simulink model "LQR_Kalman_Hardware"  (R2018b)
settings: Solver=FixedStepAuto  StartTime=0.0  StopTime=inf  FixedStep=0.002  RelTol=1e-3  EnableMultiTasking=on
undefined symbols (not defined in the file): HIL, K_lqr, qc_get_step_size
libraries: quarc_library x3, simulink x1, cstblocks x1
settings Model: SimulationMode=external  ExtModeTrigDuration=10000  Creator=ACSI-MLC  LastModifiedBy=ACSI-MLC
settings SolverCC: PositivePriorityOrder=on
settings RTWCC: SystemTargetFile=quarc_win64.tlc  TemplateMakefile=quarc_default_tmf  Description=QUARC Win64 Target
settings STFCustomTargetCC: TargetPreCompLibLocation=C:\PROGRA~3\QUARC\lib\2018b\win64\release  TargetLangStandard=C99 (ISO)  ConcurrentExecutionCompliant=on  GRTInterface=on  SystemTargetFile=quarc_win64.tlc
settings GRTTargetCC: TargetPreCompLibLocation=C:\PROGRA~3\QUARC\lib\2018b\win64\release  ParMdlRefBuildCompliant=off  CompOptLevelCompliant=off  CombineOutputUpdateFcns=off  MatFileLogging=off  CPPClassGenCompliant=off  GRTInterface=on  UseToolchainInfoCompliant=off  ExtMode=on  ExtModeMexFile=quarc_comm

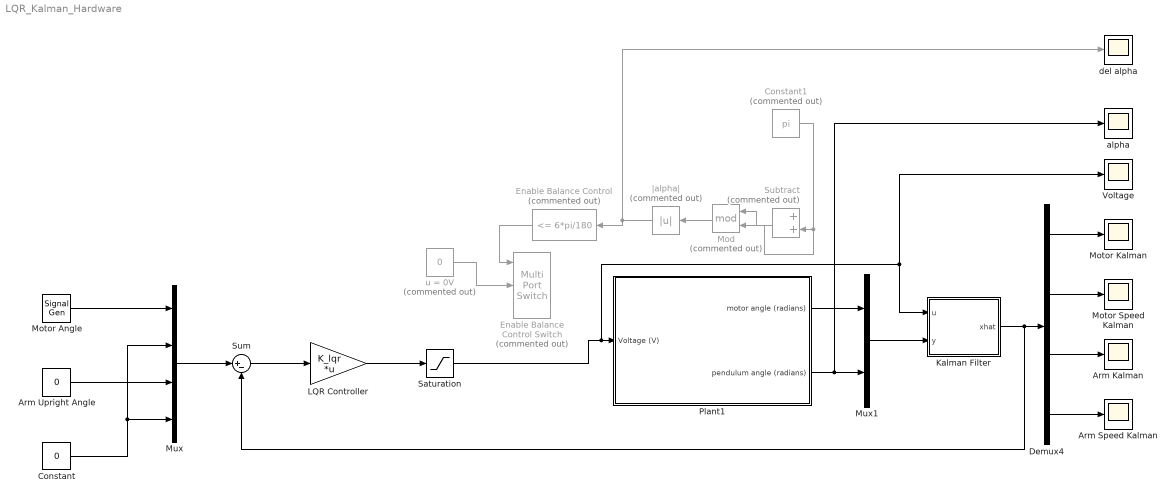
== system LQR_Kalman_Hardware ==
  Arm Kalman : Scope
  Arm Speed Kalman : Scope
  Arm Upright Angle : Constant  Value=0
  Constant : Constant  Value=0
  Constant1 : Constant  Commented=on  Value=pi
  Demux4 : Demux
  Enable Balance Control : simulink/Logic and Bit Operations/Compare To Constant  Commented=on  relop=<=  const=6*pi/180  OutDataTypeStr=uint8  ZeroCross=off
  Enable Balance Control Switch : MultiPortSwitch  Commented=on  DataPortOrder=Zero-based contiguous  Inputs=2  zeroidx=on
  Kalman Filter : Subsystem
  LQR Controller : Gain  Gain=K_lqr  Multiplication=Matrix(K*u) (u vector)
  Mod : Math  Commented=on  Operator=mod  SaturateOnIntegerOverflow=on
  Motor Angle : SignalGenerator  WaveForm=square  Amplitude=10/180*pi  Frequency=0.2
  Motor Kalman : Scope
  Motor Speed Kalman : Scope
  Mux : Mux
  Mux1 : Mux  Inputs=2
  Plant1 : Subsystem
  Saturation : Saturate  UpperLimit=18  LowerLimit=-18
  Subtract : Sum  Commented=on
  Sum : Sum  Inputs=|+-
  Voltage : Scope
  alpha : Scope
  del alpha : Scope
  u = 0V : Constant  Commented=on  Value=0
  |alpha| : Abs  Commented=on
  wires:
  u = 0V/1 -> Enable Balance Control Switch/2
  Enable Balance Control/1 -> Enable Balance Control Switch/1
  Demux4/1 -> Motor Kalman/1
  Kalman Filter/1(xhat) -> Sum/2, Demux4/1
  Mux1/1 -> Kalman Filter/2(y)
  |alpha|/1 -> Enable Balance Control/1, del alpha/1
  Sum/1 -> LQR Controller/1
  Plant1/1(motor angle (radians)) -> Mux1/1
  LQR Controller/1 -> Saturation/1
  Constant/1 -> Mux/4, Mux/2
  Demux4/4 -> Arm Speed Kalman/1
  Plant1/2(pendulum angle (radians)) -> alpha/1, Mux1/2
  Arm Upright Angle/1 -> Mux/3
  Demux4/3 -> Arm Kalman/1
  Motor Angle/1 -> Mux/1
  Demux4/2 -> Motor Speed Kalman/1
  Mux/1 -> Sum/1
  Constant1/1 -> Subtract/2, Mod/2
  Mod/1 -> |alpha|/1
  Subtract/1 -> Mod/1
  Saturation/1 -> Voltage/1, Kalman Filter/1(u), Plant1/1(Voltage (V))

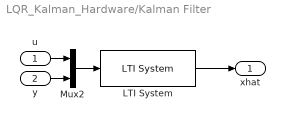
== system LQR_Kalman_Hardware/Kalman Filter ==
  u : Inport
  y : Inport  Port=2
  LTI System : cstblocks/LTI System  sys=obs_kf  IC=[0, 0, 0, 0]
  Mux2 : Mux  Inputs=2
  xhat : Outport  VectorParamsAs1DForOutWhenUnconnected=on
  wires:
  Mux2/1 -> LTI System/1
  LTI System/1 -> xhat/1
  y/1 -> Mux2/2
  u/1 -> Mux2/1

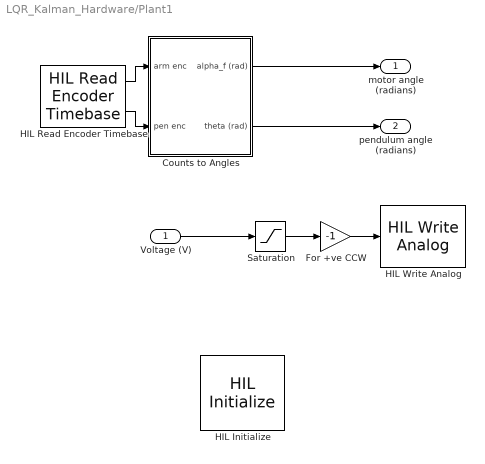
== system LQR_Kalman_Hardware/Plant1 ==
  Voltage (V) : Inport
  Counts to Angles : Subsystem
  For +ve CCW : Gain  Gain=-1
  HIL Initialize : quarc_library/Data Acquisition/Generic/Configuration/HIL Initialize  object_name=HIL-2  board_type=qube_servo2_usb  board_number=0  board_options=""  exclusive=off  active=off  hardware_clocks=[0]  clock_modes=[]  initial_clock_frequencies=[]  set_clock_params_at_start=off  set_clock_params_at_switch_in=off  set_clock_frequencies_at_start=off  set_clock_frequencies_at_switch_in=off  analog_input_channels=[0]  analog_input_configurations=[]  analog_input_maximums=3  analog_input_minimums=-3  set_analog_input_params_at_start=off  set_analog_input_params_at_switch_in=off  analog_output_channels=[0]  analog_output_maximums=15  analog_output_minimums=-15  initial_analog_outputs=[0]  final_analog_outputs=[0]  watchdog_analog_outputs=0  set_analog_output_params_at_start=off  set_analog_output_params_at_switch_in=off  set_analog_outputs_at_start=on  set_analog_outputs_at_switch_in=off  set_analog_outputs_at_terminate=on  set_analog_outputs_at_switch_out=off  set_analog_outputs_on_watchdog=on  digital_input_channels=[]  digital_output_channels=[0]  digital_output_configuration=[]  initial_digital_outputs=[1]  final_digital_outputs=[0]  watchdog_digital_outputs=[0]  set_digital_output_params_at_start=off  set_digital_output_params_at_switch_in=off  set_digital_outputs_at_start=on  set_digital_outputs_at_switch_in=off  set_digital_outputs_at_terminate=on  set_digital_outputs_at_switch_out=off  set_digital_outputs_on_watchdog=on  encoder_channels=[0:1]  quadrature=[4]  encoder_filter_frequency=[]  initial_encoder_counts=[0]  set_encoder_params_at_start=off  set_encoder_params_at_switch_in=off  set_encoder_counts_at_start=on  set_encoder_counts_at_switch_in=off  pwm_channels=[]  pwm_modes=[]  pwm_frequency=[]  pwm_configuration=[]  pwm_alignment=[]  pwm_polarity=[]  pwm_leading_deadband=[]  pwm_trailing_deadband=[]  initial_pwm_outputs=[]  final_pwm_outputs=[]  watchdog_pwm_outputs=[]  set_pwm_params_at_start=off  set_pwm_params_at_switch_in=off  set_pwm_outputs_at_start=off  set_pwm_outputs_at_switch_in=off  set_pwm_outputs_at_terminate=off  set_pwm_outputs_at_switch_out=off  set_pwm_outputs_on_watchdog=off  other_output_channels=[11000:11002]  initial_other_outputs=[0 1 0]  final_other_outputs=[1 0 0]  watchdog_other_outputs=[0 0 1]  set_other_outputs_at_start=on  set_other_outputs_at_switch_in=off  set_other_outputs_at_terminate=on  set_other_outputs_at_switch_out=off  set_other_outputs_on_watchdog=on
  HIL Read Encoder Timebase : quarc_library/Data Acquisition/Generic/Timebases/HIL Read Encoder Timebase  object_name=HIL-2  clock=0  channels=[0:1]  samples_in_buffer=max(ceil(1/qc_get_step_size), 1)  active=on  vector_output=off  data_type_mode=Inherit via back propagation  data_type=double
  HIL Write Analog : quarc_library/Data Acquisition/Generic/Immediate I//O/HIL Write Analog  object_name=HIL-2  channels=0  sample_time=-1  active=off  vector_input=off
  Saturation : Saturate  UpperLimit=10  LowerLimit=-10
  motor angle (radians) : Outport
  pendulum angle (radians) : Outport  Port=2
  wires:
  Counts to Angles/2(theta (rad)) -> pendulum angle (radians)/1
  Counts to Angles/1(alpha_f (rad)) -> motor angle (radians)/1
  HIL Read Encoder Timebase/2 -> Counts to Angles/2(pen enc)
  HIL Read Encoder Timebase/1 -> Counts to Angles/1(arm enc)
  Voltage (V)/1 -> Saturation/1
  Saturation/1 -> For +ve CCW/1
  For +ve CCW/1 -> HIL Write Analog/1

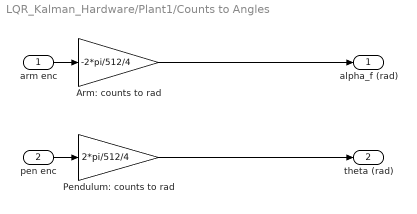
== system LQR_Kalman_Hardware/Plant1/Counts to Angles ==
  arm enc : Inport
  pen enc : Inport  Port=2
  Arm: counts to rad : Gain  Gain=-2*pi/512/4
  Pendulum: counts to rad : Gain  Gain=2*pi/512/4
  alpha_f (rad) : Outport
  theta (rad) : Outport  Port=2
  wires:
  pen enc/1 -> Pendulum: counts to rad/1
  arm enc/1 -> Arm: counts to rad/1
  Pendulum: counts to rad/1 -> theta (rad)/1
  Arm: counts to rad/1 -> alpha_f (rad)/1
